simulink model "model"  (R2017a)
settings: Solver=VariableStepAuto  StartTime=0.0  StopTime=35  RelTol=1e-3
libraries: fl_lib x5, nesl_utility x4, fuzblock x1
settings Model: Creator=mn  LastModifiedBy=mn

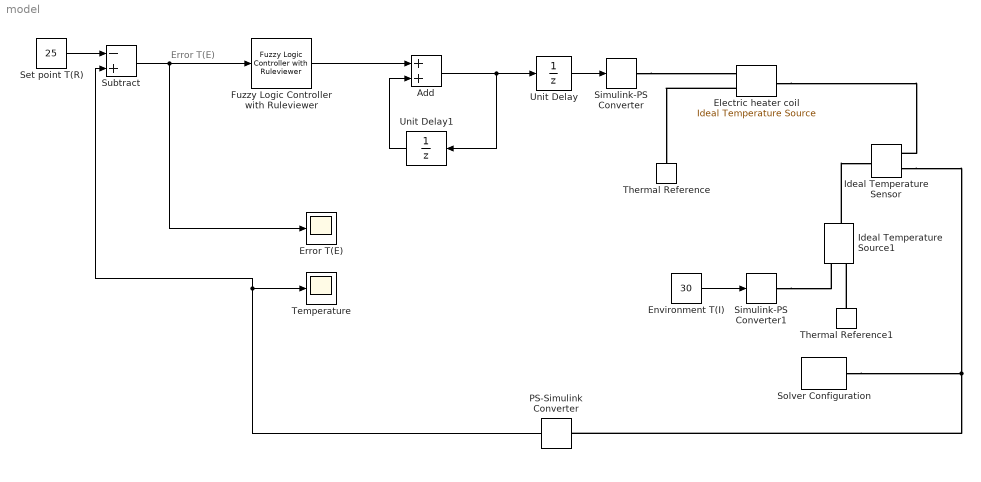
== system model ==
  note: Error T(E)
  Add : Sum
  Electric heater coil : fl_lib/Thermal/Thermal Sources/Ideal Temperature Source
      settings: SourceProductName=Simscape  SourceProductBaseCode=SS
  Environment T(I) : Constant  Value=30
  Error T(E) : Scope
  Fuzzy Logic Controller with Ruleviewer : fuzblock/Fuzzy Logic  Controller  with Ruleviewer  fismatrix=FIS  Ts=2
  Ideal Temperature Sensor : fl_lib/Thermal/Thermal Sensors/Ideal Temperature Sensor
      settings: SourceProductName=Simscape  SourceProductBaseCode=SS
  Ideal Temperature Source1 : fl_lib/Thermal/Thermal Sources/Ideal Temperature Source
      settings: SourceProductName=Simscape  SourceProductBaseCode=SS
  PS-Simulink Converter : nesl_utility/PS-Simulink Converter  PhysicalDomain=network_engine_domain  SubClassName=ps_output  LeftPortType=input  RightPortType=output  PseudoPeriodic=off  Frequencies=[]  Unit=1  AffineConversion=off
  Set point T(R) : Constant  Value=25
  Simulink-PS Converter : nesl_utility/Simulink-PS Converter  PhysicalDomain=network_engine_domain  SubClassName=ps_input  LeftPortType=input  RightPortType=output  PseudoPeriodic=off  Frequencies=[]  NoiseDistribution=none  NoiseParameters=[]  Unit=1  AffineConversion=off  FilteringAndDerivatives=provide  SimscapeFilterOrder=1  InputFilterTimeConstant=0.001  UdotUserProvided=0
  Simulink-PS Converter1 : nesl_utility/Simulink-PS Converter  PhysicalDomain=network_engine_domain  SubClassName=ps_input  LeftPortType=input  RightPortType=output  PseudoPeriodic=off  Frequencies=[]  NoiseDistribution=none  NoiseParameters=[]  Unit=1  AffineConversion=off  FilteringAndDerivatives=provide  SimscapeFilterOrder=1  InputFilterTimeConstant=0.001  UdotUserProvided=0
  Solver Configuration : nesl_utility/Solver Configuration  PhysicalDomain=network_engine_domain  SubClassName=solver  LeftPortType=input  RightPortType=generic  Accelerate=off  Tones=[]  Harmonics=[]  SimulateNoise=off  Profile=off  UseLocalSampling=off  EnableSwitchedLinearOptims=on  FrequencyDomain=off  UseCCode=off  RelTol=0.001  AbsTol=1e-06  MinStep=1e-09  ToWorkspace=off  RevertToSquareIcSolve=off  NumHomotopyIterations=100  PhasorMode=off  PhasorModeNumHarmonics=1  OverrideAbsTol=off  DoDC=off  ResidualTolerance=1e-09  UseLocalSolver=off  LocalSolverChoice=NE_BACKWARD_EULER_ADVANCER  LocalSolverSampleTime=0.001  DoFixedCost=off  MaxNonlinIter=3  MaxModeIter=2  LinearAlgebra=Sparse  DelaysMemoryBudget=1024  AutomaticFiltering=on  FilteringTimeConstant=0.001
  Subtract : Sum  Inputs=-+
  Temperature : Scope
  Thermal Reference : fl_lib/Thermal/Thermal Elements/Thermal Reference
  Thermal Reference1 : fl_lib/Thermal/Thermal Elements/Thermal Reference
  Unit Delay : UnitDelay  SampleTime=-1
  Unit Delay1 : UnitDelay  SampleTime=-1
  wires:
  Set point T(R)/1 -> Subtract/1
  Add/1 -> Unit Delay1/1, Unit Delay/1
  Unit Delay1/1 -> Add/2
  Subtract/1 -> Error T(E)/1, Fuzzy Logic Controller with Ruleviewer/1
  Unit Delay/1 -> Simulink-PS Converter/1
  PS-Simulink Converter/1 -> Subtract/2, Temperature/1
  Fuzzy Logic Controller with Ruleviewer/1 -> Add/1
  Environment T(I)/1 -> Simulink-PS Converter1/1
  connections:
  Thermal Reference1/LConn1 -- Ideal Temperature Source1/RConn2
  Simulink-PS Converter/RConn1 -- Electric heater coil/RConn1
  Electric heater coil/RConn2 -- Thermal Reference/LConn1
  Ideal Temperature Source1/LConn1 -- Ideal Temperature Sensor/LConn1
  Electric heater coil/LConn1 -- Ideal Temperature Sensor/RConn1
  Simulink-PS Converter1/RConn1 -- Ideal Temperature Source1/RConn1
  Ideal Temperature Sensor/RConn2 -- PS-Simulink Converter/LConn1 -- Solver Configuration/RConn1
